simulink model "Problem_3PI"  (R2020a)
settings: Solver=VariableStepAuto  StartTime=0.0  StopTime=10.0  RelTol=1e-3
model workspace (MAT data in the model file):
  b = Simulink.Parameter
  b.Value = 50
  b.DataType = 'auto'
  b.Dimensions = [1 1]
  ki = Simulink.Parameter
  ki.Value = 40
  ki.DataType = 'auto'
  ki.Dimensions = [1 1]
  kp = Simulink.Parameter
  kp.Value = 800
  kp.DataType = 'auto'
  kp.Dimensions = [1 1]
  m = Simulink.Parameter
  m.Value = 1000
  m.DataType = 'auto'
  m.Dimensions = [1 1]
settings Model: Creator=hp  LastModifiedBy=hp

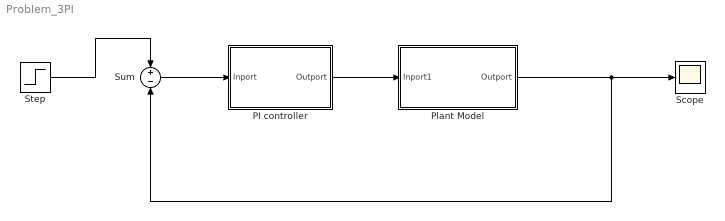
== system Problem_3PI ==
  PI controller : Subsystem
  Plant Model : Subsystem
  Scope : Scope
  Step : Step  SampleTime=0
  Sum : Sum  Inputs=+-
  wires:
  PI controller/1(Outport) -> Plant Model/1(Inport1)
  Plant Model/1(Outport) -> Sum/2, Scope/1
  Step/1 -> Sum/1
  Sum/1 -> PI controller/1(Inport)

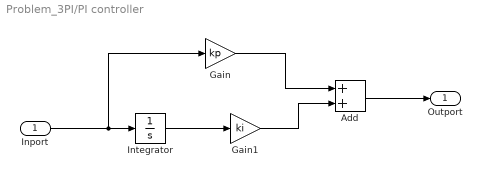
== system Problem_3PI/PI controller ==
  Inport : Inport
  Add : Sum
  Gain : Gain  Gain=kp
  Gain1 : Gain  Gain=ki
  Integrator : Integrator
  Outport : Outport
  wires:
  Inport/1 -> Gain/1, Integrator/1
  Add/1 -> Outport/1
  Integrator/1 -> Gain1/1
  Gain1/1 -> Add/2
  Gain/1 -> Add/1

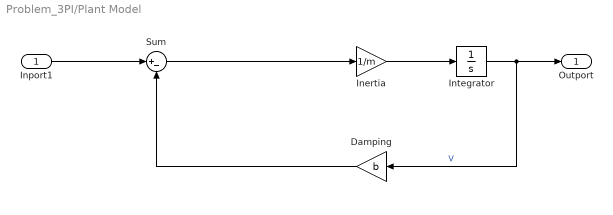
== system Problem_3PI/Plant Model ==
  Inport1 : Inport
  Damping : Gain  Gain=b
  Inertia : Gain  Gain=1/m
  Integrator : Integrator
  Sum : Sum  Inputs=|+-
  Outport : Outport
  wires:
  Integrator/1 -> Outport/1, Damping/1  "V"
  Inport1/1 -> Sum/1
  Sum/1 -> Inertia/1
  Inertia/1 -> Integrator/1
  Damping/1 -> Sum/2
